simulink model "multiportswitch_basic"  (Simulink 7.9)
settings: Solver=FixedStepDiscrete  StartTime=0.0  StopTime=10.0  FixedStep=1  RelTol=1e-3
settings Model: Creator=Nyenyec  LastModifiedBy=hnine
settings OptimizationCC: InitFltsAndDblsToZero=on
settings DebuggingCC: SaveWithParameterizedLinksMsg=none  FcnCallInpInsideContextMsg=Use local settings  StrictBusMsg=Warning
settings SFSimCC: SimParseCustomCode=off
settings GRTTargetCC: TargetFcnLib=ansi_tfl_tmw.mat  CombineOutputUpdateFcns=off  GRTInterface=on

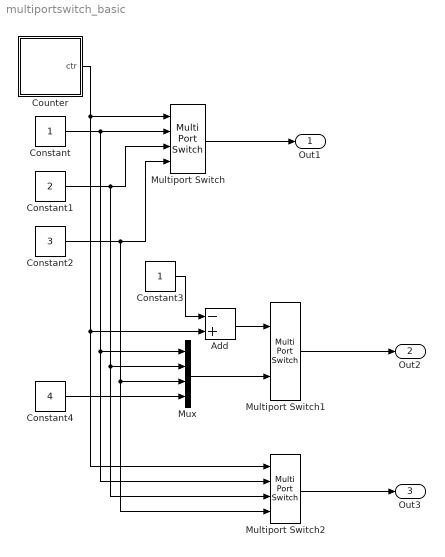
== system multiportswitch_basic ==
  Add : Sum  Inputs=-+
  Constant : Constant
  Constant1 : Constant  Value=2
  Constant2 : Constant  Value=3
  Constant3 : Constant
  Constant4 : Constant  Value=4
  Counter : Stateflow chart  TreatAsAtomicUnit=on
  Multiport Switch : MultiPortSwitch  DiagnosticForDefault=None  zeroidx=off
  Multiport Switch1 : MultiPortSwitch  DataPortOrder=Zero-based contiguous  Inputs=1  zeroidx=on
  Multiport Switch2 : MultiPortSwitch  DataPortOrder=Specify indices  DataPortIndices={[2,1],3}  DataPortForDefault=Additional data port  DiagnosticForDefault=None  zeroidx=off
  Mux : Mux
  Out1 : Outport
  Out2 : Outport  Port=2
  Out3 : Outport  Port=3
  wires:
  Counter/1(ctr) -> Multiport Switch/1, Add/2, Multiport Switch2/1
  Constant/1 -> Multiport Switch/2, Multiport Switch2/2, Mux/1
  Constant1/1 -> Multiport Switch/3, Multiport Switch2/3, Mux/2
  Constant2/1 -> Multiport Switch/4, Multiport Switch2/4, Mux/3
  Multiport Switch/1 -> Out1/1
  Multiport Switch1/1 -> Out2/1
  Mux/1 -> Multiport Switch1/2
  Add/1 -> Multiport Switch1/1
  Constant3/1 -> Add/1
  Multiport Switch2/1 -> Out3/1
  Constant4/1 -> Mux/4

== stateflow chart Counter ==
  settings: executeAtInitialization=1
  state s1
  (default) -> s1
  s1 -> s1 [order 1] : [ctr < 4] / ctr = ctr+1;
  s1 -> s1 [order 2] : [ctr >= 4] / ctr = 1;
  data: ctr output double =1
